simulink model "lab5_cascada"  (R2023b)
settings: Solver=ode45  StartTime=0.0  StopTime=400  RelTol=1e-3
settings Model: Creator=Daniela  LastModifiedBy=Daniela

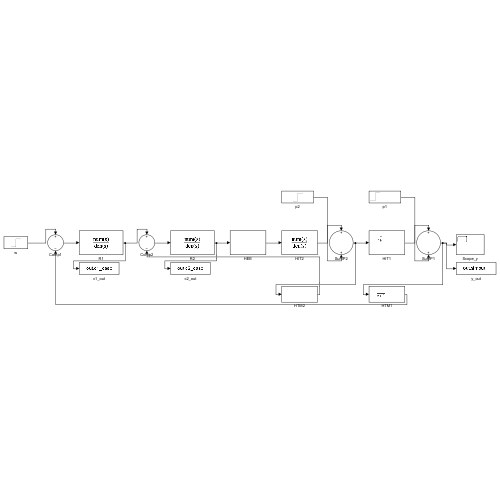
[thumbnail: Simulink's stored preview of the top-level diagram]
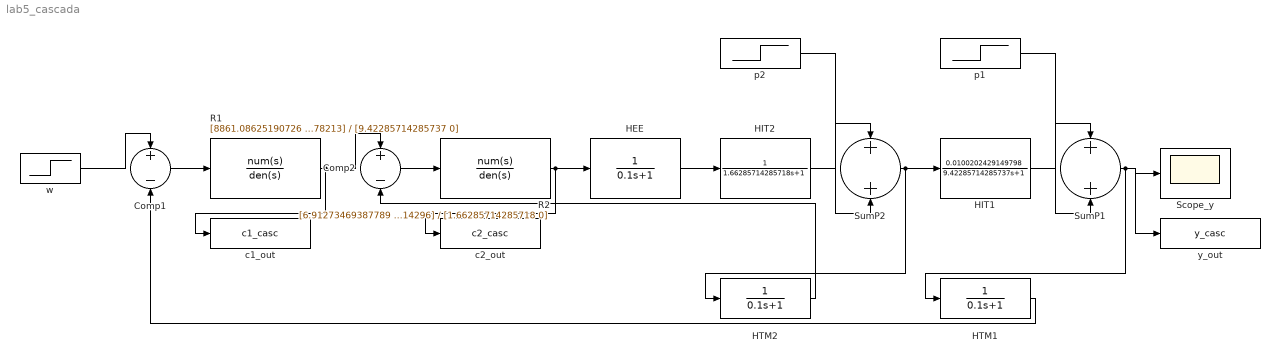
== system lab5_cascada ==
  Comp1 : Sum  Inputs=+-
  Comp2 : Sum  Inputs=+-
  HEE : TransferFcn  Numerator=1  Denominator=[0.1 1]
  HIT1 : TransferFcn  Numerator=0.0100202429149798  Denominator=[9.42285714285737 1]
  HIT2 : TransferFcn  Numerator=1  Denominator=[1.66285714285718 1]
  HTM1 : TransferFcn  Numerator=1  Denominator=[0.1 1]
  HTM2 : TransferFcn  Numerator=1  Denominator=[0.1 1]
  R1 : TransferFcn  Numerator=[8861.08625190726 940.38210678213]  Denominator=[9.42285714285737 0]
  R2 : TransferFcn  Numerator=[6.91273469387789 4.15714285714296]  Denominator=[1.66285714285718 0]
  Scope_y : Scope
  SumP1 : Sum
  SumP2 : Sum
  c1_out : ToWorkspace  VariableName=c1_casc  SampleTime=-1
  c2_out : ToWorkspace  VariableName=c2_casc  SampleTime=-1
  p1 : Step  Time=0  After=0  SampleTime=0
  p2 : Step  Time=80  SampleTime=0
  w : Step  Time=0  After=0.1  SampleTime=0
  y_out : ToWorkspace  VariableName=y_casc  SampleTime=-1
  wires:
  w/1 -> Comp1/1
  Comp1/1 -> R1/1
  R1/1 -> Comp2/1, c1_out/1
  Comp2/1 -> R2/1
  R2/1 -> HEE/1, c2_out/1
  HEE/1 -> HIT2/1
  HIT2/1 -> SumP2/1
  p2/1 -> SumP2/2
  SumP2/1 -> HIT1/1, HTM2/1
  HIT1/1 -> SumP1/1
  p1/1 -> SumP1/2
  SumP1/1 -> Scope_y/1, y_out/1, HTM1/1
  HTM1/1 -> Comp1/2
  HTM2/1 -> Comp2/2
